simulink model "probOne"  (R2020b)
settings: Solver=ode45  StartTime=0.0  StopTime=30.0  MaxStep=0.002  RelTol=1e-3
model workspace (MAT data in the model file):
  b = Simulink.Parameter
  b.Value = 50
  b.DataType = 'auto'
  b.Dimensions = [1 1]
  k1 = Simulink.Parameter
  k1.Value = 50
  k1.DataType = 'auto'
  k1.Dimensions = [1 1]
  k12 = Simulink.Parameter
  k12.Value = 59718.75
  k12.DataType = 'auto'
  k12.Dimensions = [1 1]
  m1 = Simulink.Parameter
  m1.Value = 100
  m1.DataType = 'auto'
  m1.Dimensions = [1 1]
  m2 = Simulink.Parameter
  m2.Value = 599.455357143
  m2.DataType = 'auto'
  m2.Dimensions = [1 1]
settings Model: Creator='Z'ome  LastModifiedBy='Z'ome

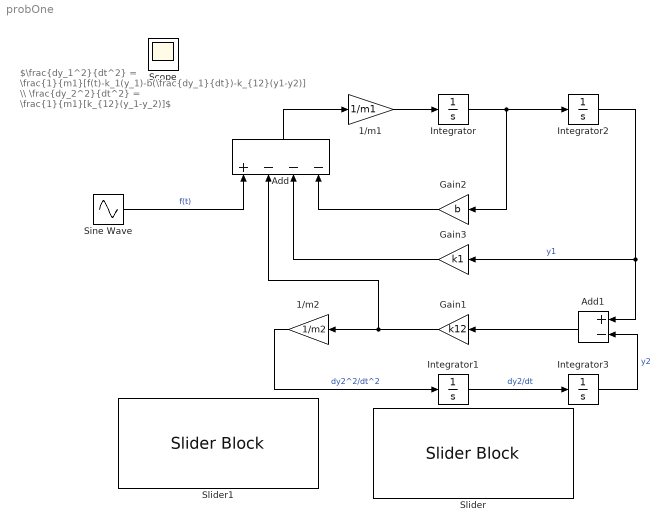
== system probOne ==
  note: $\frac{dy_1^2}{dt^2} = \frac{1}{m1}[f(t)-k_1(y_1)-b(\frac{dy_1}{dt})-k_{12}(y1-y2)] \\ \frac{dy_2^2}{dt^2} = \frac{1}{m1}[k_{12}(y_1-y_2)]$
  1/m1 : Gain  Gain=1/m1
  1/m2 : Gain  Gain=1/m2
  Add : Sum  Inputs=+---
  Add1 : Sum  Inputs=+-
  Gain1 : Gain  Gain=k12
  Gain2 : Gain  Gain=b
  Gain3 : Gain  Gain=k1
  Integrator{,1..3} (4 alike) : Integrator
  Sine Wave : Sin  Amplitude=2  Frequency=10  SampleTime=0
  Slider : SliderBlock  ScaleMin=50000  ScaleMax=100000
  Slider1 : SliderBlock  ScaleMin=500  ScaleMax=800
  Scope : Scope
  wires:
  Integrator1/1 -> Integrator3/1  "dy2/dt"
  Integrator/1 -> Gain2/1, Integrator2/1
  Integrator3/1 -> Add1/2  "y2"
  Integrator2/1 -> Gain3/1, Add1/1  "y1"
  Add1/1 -> Gain1/1
  Gain1/1 -> Add/2, 1/m2/1
  1/m2/1 -> Integrator1/1  "dy2^2/dt^2"
  1/m1/1 -> Integrator/1
  Gain2/1 -> Add/4
  Gain3/1 -> Add/3
  Sine Wave/1 -> Add/1  "f(t)"
  Add/1 -> 1/m1/1
